simulink model "gm_uz_ssi_interface_2025b"  (R2025b)
settings: Solver=FixedStepDiscrete  StartTime=0.0  StopTime=0.005  RelTol=1e-3
undefined symbols (not defined in the file or in its folder): binary_or_gray, bit_sum, delay_first_clk_on_off, f_ADC, f_clock, PLL, ssi_clk_divider, ssi_encoder_bit_width_multi_turn, ssi_encoder_bit_width_single_turn, ssi_encoder_number_of_status_bits, t_ADC, t_clock, XData
libraries: hdlmdlgenlib x104, hdlsllib x90, simulink x33, simulink_extras x7
(part 1 of 4)
settings Model: Creator=micha  LastModifiedBy=micha
settings SolverCC: AlgebraicLoopSolver=TrustRegion
settings DataIOCC: LimitDataPoints=on  SaveOutput=off  SaveTime=off
settings OptimizationCC: BlockReduction=off  ConditionallyExecuteInputs=off  DefaultParameterBehavior=Inlined  InheritOutputTypeSmallerThanSingle=on  LifeSpan=inf
settings DebuggingCC: AlgebraicLoopMsg=error  ArtificialAlgebraicLoopMsg=none  InheritedTsInSrcMsg=none  SingleTaskRateTransMsg=error  UnconnectedInputMsg=warning  UnconnectedOutputMsg=warning  UnconnectedLineMsg=warning  AllowSymbolicDim=off  StrictBusMsg=ErrorOnBusTreatedAsVector  SFUnexpectedBacktrackingDiag=warning  SFNoUnconditionalDefaultTransitionDiag=warning  SFExecutionAtInitializationDiag=none  ArithmeticOperatorsInVariantConditions=warning
settings HardwareCC: ProdBitPerPointer=32.0  ProdBitPerSizeT=32.0  ProdBitPerPtrDiffT=32.0  ProdLargestAtomicFloat=None  ProdIntDivRoundTo=Undefined  ProdEndianess=Unspecified  ProdWordSize=32.0  ProdHWDeviceType=ASIC/FPGA->ASIC/FPGA  ProdEqTarget=off
settings ModelReferenceCC: EnableRefExpFcnMdlSchedulingChecks=on
settings SFSimCC: SimUseLocalCustomCode=off  CustomCodeUndefinedFunction=UseInterfaceOnly
settings RTWCC: RTWUseLocalCustomCode=off  GPUComputeCapability=3.5  DLArmComputeVersion=19.05
settings CodeAppCC: StateflowObjectComments=on
settings GRTTargetCC: TargetLangStandard=C89/C90 (ANSI)
settings ConfigComp: CovScope=ReferencedModels  CovMetricSettings=dw  CovSaveCumulativeToWorkspaceVar=on  CovSaveSingleToWorkspaceVar=on  CovExternalEMLEnable=off  CovSFcnEnable=off

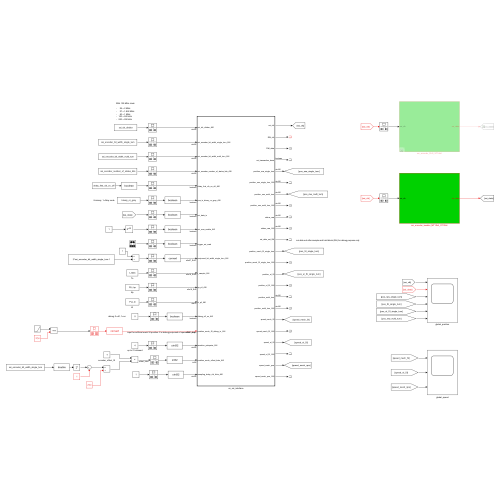
[thumbnail: Simulink's stored preview of the top-level diagram]
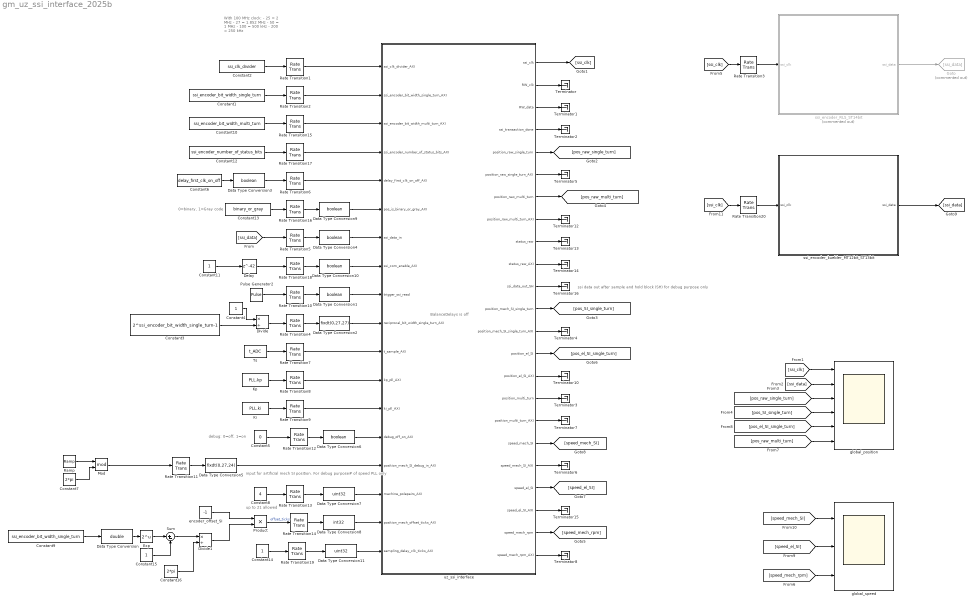
== system gm_uz_ssi_interface_2025b ==
  note: 0=binary, 1=Gray code
  note: With 100 MHz clock:
      |
      | -     25 = 2 MHz
      | -     27 = 1.852 MHz
      | -     50 = 1 MHz
      | -   100 = 500 kHz
      | -   200 = 250 kHz
  note: BalanceDelays is off
  note: debug: 0=off, 1=on
  note: up to 21 allowed
  note: ssi data out after sample and hold block (SH) for debug purpose only
  note: input for artificial mech SI position. For debug purpose# of speed PLL only
  Constant1 : Constant  Value=ssi_encoder_bit_width_single_turn  OutDataTypeStr=uint32  SampleTime=t_clock
  Constant10 : Constant  Value=ssi_encoder_bit_width_multi_turn  OutDataTypeStr=uint32  SampleTime=t_clock
  Constant{4,11,14..15} (4 alike) : Constant  SampleTime=t_clock
  Constant12 : Constant  Value=ssi_encoder_number_of_status_bits  OutDataTypeStr=uint32  SampleTime=t_clock
  Constant13 : Constant  Value=binary_or_gray  OutDataTypeStr=uint32  SampleTime=t_clock
  Constant16 : Constant  Value=2*pi  SampleTime=t_clock
  Constant2 : Constant  Value=ssi_clk_divider  OutDataTypeStr=uint32  SampleTime=t_clock
  Constant3 : Constant  Value=2^ssi_encoder_bit_width_single_turn-1  OutDataTypeStr=double  SampleTime=t_clock
  Constant5 : Constant  Value=0  SampleTime=t_clock
  Constant6 : Constant  Value=delay_first_clk_on_off  OutDataTypeStr=uint32  SampleTime=t_clock
  Constant7 : Constant  Value=2*pi  SampleTime=t_clock
  Constant8 : Constant  Value=4  SampleTime=t_clock
  Constant9 : Constant  Value=ssi_encoder_bit_width_single_turn  OutDataTypeStr=uint32  SampleTime=t_clock
  Data Type Conversion : DataTypeConversion  OutDataTypeStr=double  SaturateOnIntegerOverflow=off  RndMeth=Floor
  Data Type Conversion{1,3..4,6,9..10} (6 alike) : DataTypeConversion  OutDataTypeStr=boolean  SaturateOnIntegerOverflow=off  RndMeth=Floor
  Data Type Conversion11 : DataTypeConversion  OutDataTypeStr=uint32  SaturateOnIntegerOverflow=off  RndMeth=Floor
  Data Type Conversion2 : DataTypeConversion  OutDataTypeStr=fixdt(0,27,27)  SaturateOnIntegerOverflow=off  RndMeth=Floor
  Data Type Conversion5 : DataTypeConversion  OutDataTypeStr=fixdt(0,27,24)  SaturateOnIntegerOverflow=off  RndMeth=Floor
  Data Type Conversion7 : DataTypeConversion  OutDataTypeStr=uint32  SaturateOnIntegerOverflow=off  RndMeth=Floor
  Data Type Conversion8 : DataTypeConversion  OutDataTypeStr=int32  SaturateOnIntegerOverflow=off  RndMeth=Floor
  Delay : Delay  DelayLength=42
  Divide : Product  Inputs=*/
  Divide1 : Product  Inputs=*/
  Exp : Math  Operator=2^u
  Goto : Goto  Commented=on  GotoTag=ssi_data
  Ki : Constant  Value=PLL.ki  OutDataTypeStr=fixdt(0,18,0)  SampleTime=-1
  Kp : Constant  Value=PLL.kp  OutDataTypeStr=fixdt(0,18,5)  SampleTime=-1
  Mod : Math  Operator=mod
  Product : Product
  Pulse Generator2 : DiscretePulseGenerator  Period=f_clock/f_ADC  PulseWidth=0.04*f_clock/f_ADC  PhaseDelay=250  SampleTime=t_clock
  Ramp : simulink/Sources/Ramp  slope=2*pi*100  start=7.5e-5  InitialOutput=0
  Rate Transition{1..20} (20 alike) : RateTransition  OutPortSampleTime=t_clock
  Sum : Sum  Inputs=|+-
  Terminator{,1..8,10,12..16} (15 alike) : Terminator
  Ts : Constant  Value=t_ADC  OutDataTypeStr=fixdt(0,18,24)  SampleTime=-1
  encoder_offset_SI : Constant  Value=-1  SampleTime=t_clock
  global_position : Scope  NumInputPorts=6
      settings: ActiveDisplayYMinimum=-0.125  ActiveDisplayYMaximum=1.125  DataLoggingVariableName=ScopeData2
  global_speed : Scope  NumInputPorts=3
      settings: ActiveDisplayYMinimum=-40.08166  ActiveDisplayYMaximum=351.59007
  ssi_encoder_RLS_ST14bit : Subsystem  Commented=on
  ssi_encoder_kuebler_MT12bit_ST13bit : Subsystem
  uz_ssi_interface : Subsystem  TreatAsAtomicUnit=on
  wires:
  Data Type Conversion/1 -> Exp/1
  Divide1/1 -> Product/2
  Constant16/1 -> Divide1/2
  Sum/1 -> Divide1/1
  Exp/1 -> Sum/1
  Constant15/1 -> Sum/2
  Constant9/1 -> Data Type Conversion/1
  Product/1 -> Rate Transition14/1  "offset_ticks"
  uz_ssi_interface/17(position_multi_turn_AXI) -> Terminator7/1
  uz_ssi_interface/16(position_multi_turn) -> Terminator3/1
  ssi_encoder_kuebler_MT12bit_ST13bit/1(ssi_data) -> [ssi_data]
  Rate Transition20/1 -> ssi_encoder_kuebler_MT12bit_ST13bit/1(ssi_clk)
  [ssi_clk] -> Rate Transition20/1
  Constant14/1 -> Rate Transition19/1
  Rate Transition19/1 -> Data Type Conversion11/1
  Data Type Conversion11/1 -> uz_ssi_interface/18(sampling_delay_clk_ticks_AXI)
  [speed_el_SI] -> global_speed/2
  [speed_mech_SI] -> global_speed/1
  [pos_el_SI_single_turn] -> global_position/5
  [pos_raw_multi_turn] -> global_position/6
  [speed_mech_rpm] -> global_speed/3
  [ssi_clk] -> Rate Transition3/1
  Delay/1 -> Rate Transition18/1
  uz_ssi_interface/22(speed_mech_rpm) -> [speed_mech_rpm]
  uz_ssi_interface/11(ssi_data_out_SH) -> Terminator16/1
  uz_ssi_interface/12(position_mech_SI_single_turn) -> [pos_SI_single_turn]
  [pos_SI_single_turn] -> global_position/4
  [pos_raw_single_turn] -> global_position/3
  uz_ssi_interface/5(position_raw_single_turn) -> [pos_raw_single_turn]
  [ssi_data] -> global_position/2
  [ssi_clk] -> global_position/1
  uz_ssi_interface/20(speed_el_SI) -> [speed_el_SI]
  uz_ssi_interface/21(speed_el_SI_AXI) -> Terminator15/1
  uz_ssi_interface/10(status_raw_AXI) -> Terminator14/1
  uz_ssi_interface/9(status_raw) -> Terminator13/1
  uz_ssi_interface/8(position_raw_multi_turn_AXI) -> Terminator12/1
  uz_ssi_interface/7(position_raw_multi_turn) -> [pos_raw_multi_turn]
  Constant11/1 -> Delay/1
  Rate Transition18/1 -> Data Type Conversion10/1
  Data Type Conversion10/1 -> uz_ssi_interface/8(ssi_com_enable_AXI)
  Constant12/1 -> Rate Transition17/1
  Rate Transition17/1 -> uz_ssi_interface/4(ssi_encoder_number_of_status_bits_AXI)
  Data Type Conversion9/1 -> uz_ssi_interface/6(pos_is_binary_or_gray_AXI)
  Constant13/1 -> Rate Transition16/1
  Rate Transition16/1 -> Data Type Conversion9/1
  Constant10/1 -> Rate Transition15/1
  Rate Transition15/1 -> uz_ssi_interface/3(ssi_encoder_bit_width_multi_turn_AXI)
  uz_ssi_interface/15(position_el_SI_AXI) -> Terminator10/1
  uz_ssi_interface/14(position_el_SI) -> [pos_el_SI_single_turn]
  Data Type Conversion8/1 -> uz_ssi_interface/17(position_mech_offset_ticks_AXI)
  encoder_offset_SI/1 -> Product/1
  Rate Transition14/1 -> Data Type Conversion8/1
  Constant8/1 -> Rate Transition13/1
  Data Type Conversion7/1 -> uz_ssi_interface/16(machine_polepairs_AXI)
  Rate Transition13/1 -> Data Type Conversion7/1
  uz_ssi_interface/23(speed_mech_rpm_AXI) -> Terminator8/1
  Constant7/1 -> Mod/2
  Ramp/1 -> Mod/1
  Mod/1 -> Rate Transition11/1
  Constant5/1 -> Rate Transition12/1
  Rate Transition12/1 -> Data Type Conversion6/1
  Data Type Conversion6/1 -> uz_ssi_interface/14(debug_off_on_AXI)
  Data Type Conversion5/1 -> uz_ssi_interface/15(position_mech_SI_debug_in_AXI)
  Rate Transition11/1 -> Data Type Conversion5/1
  uz_ssi_interface/19(speed_mech_SI_AXI) -> Terminator6/1
  uz_ssi_interface/18(speed_mech_SI) -> [speed_mech_SI]
  Rate Transition9/1 -> uz_ssi_interface/13(ki_pll_AXI)
  Ki/1 -> Rate Transition9/1
  Rate Transition8/1 -> uz_ssi_interface/12(kp_pll_AXI)
  Kp/1 -> Rate Transition8/1
  Rate Transition7/1 -> uz_ssi_interface/11(t_sample_AXI)
  Ts/1 -> Rate Transition7/1
  uz_ssi_interface/13(position_mech_SI_single_turn_AXI) -> Terminator4/1
  Divide/1 -> Rate Transition4/1
  Constant4/1 -> Divide/1
  Data Type Conversion2/1 -> uz_ssi_interface/10(reciprocal_bit_width_single_turn_AXI)
  Rate Transition4/1 -> Data Type Conversion2/1
  Constant3/1 -> Divide/2
  Data Type Conversion4/1 -> uz_ssi_interface/7(ssi_data_in)
  Rate Transition5/1 -> Data Type Conversion4/1
  uz_ssi_interface/6(position_raw_single_turn_AXI) -> Terminator5/1
  Constant6/1 -> Data Type Conversion3/1
  Data Type Conversion3/1 -> Rate Transition6/1
  Rate Transition6/1 -> uz_ssi_interface/5(delay_first_clk_on_off_AXI)
  Data Type Conversion1/1 -> uz_ssi_interface/9(trigger_ssi_read)
  uz_ssi_interface/2(RW_clk) -> Terminator/1
  uz_ssi_interface/4(ssi_transaction_done) -> Terminator2/1
  uz_ssi_interface/3(RW_data) -> Terminator1/1
  uz_ssi_interface/1(ssi_clk) -> [ssi_clk]
  [ssi_data] -> Rate Transition5/1
  ssi_encoder_RLS_ST14bit/1(ssi_data) -> Goto/1
  Rate Transition3/1 -> ssi_encoder_RLS_ST14bit/1(ssi_clk)
  Rate Transition2/1 -> uz_ssi_interface/2(ssi_encoder_bit_width_single_turn_AXI)
  Constant1/1 -> Rate Transition2/1
  Rate Transition1/1 -> uz_ssi_interface/1(ssi_clk_divider_AXI)
  Constant2/1 -> Rate Transition1/1
  Pulse Generator2/1 -> Rate Transition10/1
  Rate Transition10/1 -> Data Type Conversion1/1

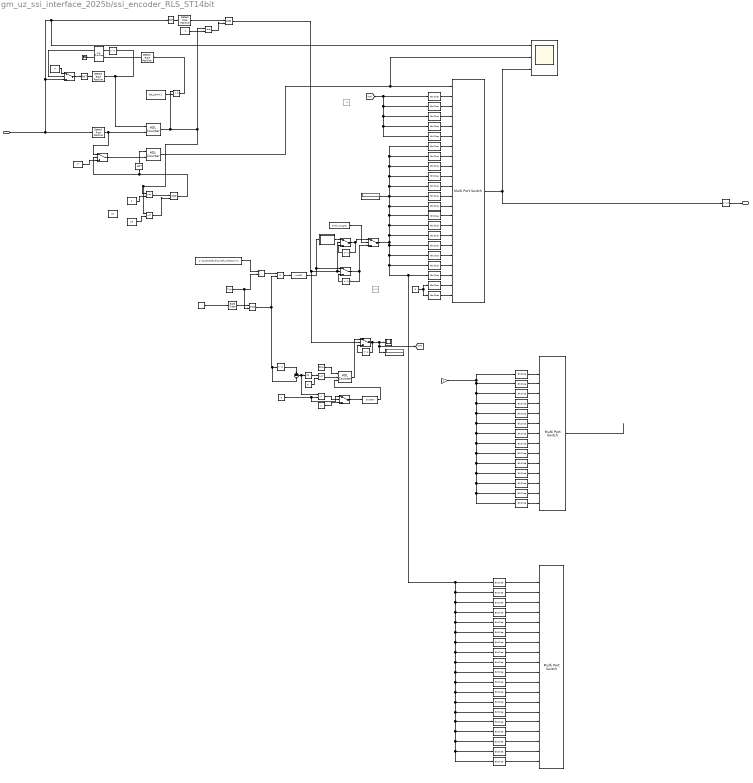
== system gm_uz_ssi_interface_2025b/ssi_encoder_RLS_ST14bit ==
  note: 19 bit single turn
  note: singleturn information
  note: Detect first falling edge of the clock
  note: 170 ns delay of the readhead
  note: multiturn information
  note: 14 bit single turn
  note: 5bit multiturn, 14bit single turn 2bit status
  ssi_clk : Inport
  AND : Logic  IconShape=distinctive  AllPortsSameDT=off  OutDataTypeStr=boolean
  AND1 : Logic  IconShape=distinctive  AllPortsSameDT=off  OutDataTypeStr=boolean
  Abs : Abs  SaturateOnIntegerOverflow=off
  Bit Slice{1,14,19,26,40} (5 alike) : hdlsllib/Logic and Bit Operations/Bit Slice  lidx=1  ridx=1
  Bit Slice10 : hdlsllib/Logic and Bit Operations/Bit Slice  lidx=5  ridx=5
  Bit Slice{11,16,23,37} (4 alike) : hdlsllib/Logic and Bit Operations/Bit Slice  lidx=4  ridx=4
  Bit Slice{12,17,24,38} (4 alike) : hdlsllib/Logic and Bit Operations/Bit Slice  lidx=3  ridx=3
  Bit Slice{13,18,25,39} (4 alike) : hdlsllib/Logic and Bit Operations/Bit Slice  lidx=2  ridx=2
  Bit Slice{15,20..21,27,41} (5 alike) : hdlsllib/Logic and Bit Operations/Bit Slice  lidx=0  ridx=0
  Bit Slice2 : hdlsllib/Logic and Bit Operations/Bit Slice  lidx=13  ridx=13
  Bit Slice22 : hdlsllib/Logic and Bit Operations/Bit Slice  lidx=5  ridx=5
  Bit Slice28 : hdlsllib/Logic and Bit Operations/Bit Slice  lidx=13  ridx=13
  Bit Slice29 : hdlsllib/Logic and Bit Operations/Bit Slice  lidx=12  ridx=12
  Bit Slice3 : hdlsllib/Logic and Bit Operations/Bit Slice  lidx=12  ridx=12
  Bit Slice30 : hdlsllib/Logic and Bit Operations/Bit Slice  lidx=11  ridx=11
  Bit Slice31 : hdlsllib/Logic and Bit Operations/Bit Slice  lidx=10  ridx=10
  Bit Slice32 : hdlsllib/Logic and Bit Operations/Bit Slice  lidx=9  ridx=9
  Bit Slice33 : hdlsllib/Logic and Bit Operations/Bit Slice  lidx=8  ridx=8
  Bit Slice34 : hdlsllib/Logic and Bit Operations/Bit Slice  lidx=7  ridx=7
  Bit Slice35 : hdlsllib/Logic and Bit Operations/Bit Slice  lidx=6  ridx=6
  Bit Slice36 : hdlsllib/Logic and Bit Operations/Bit Slice  lidx=5  ridx=5
  Bit Slice4 : hdlsllib/Logic and Bit Operations/Bit Slice  lidx=11  ridx=11
  Bit Slice42 : hdlsllib/Logic and Bit Operations/Bit Slice  lidx=13  ridx=13
  Bit Slice43 : hdlsllib/Logic and Bit Operations/Bit Slice  lidx=12  ridx=12
  Bit Slice44 : hdlsllib/Logic and Bit Operations/Bit Slice  lidx=11  ridx=11
  Bit Slice45 : hdlsllib/Logic and Bit Operations/Bit Slice  lidx=10  ridx=10
  Bit Slice46 : hdlsllib/Logic and Bit Operations/Bit Slice  lidx=9  ridx=9
  Bit Slice47 : hdlsllib/Logic and Bit Operations/Bit Slice  lidx=8  ridx=8
  Bit Slice48 : hdlsllib/Logic and Bit Operations/Bit Slice  lidx=7  ridx=7
  Bit Slice49 : hdlsllib/Logic and Bit Operations/Bit Slice  lidx=6  ridx=6
  Bit Slice5 : hdlsllib/Logic and Bit Operations/Bit Slice  lidx=10  ridx=10
  Bit Slice50 : hdlsllib/Logic and Bit Operations/Bit Slice  lidx=18  ridx=18
  Bit Slice51 : hdlsllib/Logic and Bit Operations/Bit Slice  lidx=17  ridx=17
  Bit Slice52 : hdlsllib/Logic and Bit Operations/Bit Slice  lidx=16  ridx=16
  Bit Slice53 : hdlsllib/Logic and Bit Operations/Bit Slice  lidx=15  ridx=15
  Bit Slice54 : hdlsllib/Logic and Bit Operations/Bit Slice  lidx=14  ridx=14
  Bit Slice6 : hdlsllib/Logic and Bit Operations/Bit Slice  lidx=9  ridx=9
  Bit Slice7 : hdlsllib/Logic and Bit Operations/Bit Slice  lidx=8  ridx=8
  Bit Slice8 : hdlsllib/Logic and Bit Operations/Bit Slice  lidx=7  ridx=7
  Bit Slice9 : hdlsllib/Logic and Bit Operations/Bit Slice  lidx=6  ridx=6
  Constant : Constant  Value=bit_sum+1  SampleTime=t_clock
  Constant1 : Constant  Value=0  SampleTime=t_clock
  Constant10 : Constant  Value=false  SampleTime=t_clock
  Constant11 : Constant  Value=0  SampleTime=t_clock
  Constant12 : Constant  SampleTime=t_clock
  Constant13 : Constant  Value=0  OutDataTypeStr=uint32  SampleTime=t_clock
  Constant14 : Constant  Commented=on  Value=19  OutDataTypeStr=uint32  SampleTime=t_clock
  Constant15 : Constant  Value=binary_or_gray  SampleTime=t_clock
  Constant16 : Constant  Value=15  SampleTime=t_clock
  Constant2 : Constant  SampleTime=t_clock
  Constant3 : Constant  Value=0  OutDataTypeStr=boolean  SampleTime=t_clock
  Constant4 : Constant  Value=5  SampleTime=t_clock
  Constant5 : Constant  Value=2  SampleTime=t_clock
  Constant6 : Constant  Commented=on  Value=3875  OutDataTypeStr=uint32  SampleTime=t_clock
  Constant7 : Constant  Value=2*pi  SampleTime=t_clock
  Constant8 : Constant  Value=22  SampleTime=t_clock
  Constant9 : Constant  Value=2^ssi_encoder_bit_width_single_turn-1  SampleTime=t_clock
  Data Type Conversion : DataTypeConversion  OutDataTypeStr=uint32  SaturateOnIntegerOverflow=off  RndMeth=Floor
  Data Type Conversion1 : DataTypeConversion  OutDataTypeStr=boolean  SaturateOnIntegerOverflow=off  RndMeth=Floor
  Delay : Delay  DelayLength=1
  Delay1 : Delay  DelayLength=17  SampleTime=t_clock
  Delay2 : Delay  DelayLength=1  SampleTime=t_clock
  Delay3 : Delay  DelayLength=1
  Delay4 : Delay  DelayLength=1  InitialCondition=19  SampleTime=t_clock
  Delay5 : Delay  DelayLength=1  SampleTime=t_clock
  Detect Rise Positive{,1..3} (4 alike) : simulink/Logic and Bit Operations/Detect Rise Positive  vinit=0  OutDataTypeStr=boolean
  Display : Display
  Display1 : Display
  Divide : Product  Inputs=*/
  Gain : Gain
  HDL Counter : hdlsllib/Sources/HDL Counter  CountType=Count limited  CountInit=0  CountStep=1  CountMax=bit_sum+1  CountFromType=Initial value  CountFrom=0  CountResetPort=on  CountLoadPort=off  CountEnbPort=on  CountDirPort=off  CountHitOutputPort=off  CountDataType=Unsigned  CountWordLen=8  CountFracLen=0  CountSampTime=t_clock
  HDL Counter1 : hdlsllib/Sources/HDL Counter  CountType=Count limited  CountInit=0  CountStep=1  CountMax=bit_sum+1  CountFromType=Initial value  CountFrom=0  CountResetPort=on  CountLoadPort=off  CountEnbPort=on  CountDirPort=off  CountHitOutputPort=off  CountDataType=Unsigned  CountWordLen=8  CountFracLen=0  CountSampTime=t_clock
  HDL Counter2 : hdlsllib/Sources/HDL Counter  CountType=Count limited  CountInit=19  CountStep=1  CountMax=ssi_encoder_bit_width_multi_turn  CountFromType=Initial value  CountFrom=19  CountResetPort=on  CountLoadPort=off  CountEnbPort=on  CountDirPort=on  CountHitOutputPort=off  CountDataType=Unsigned  CountWordLen=5  CountFracLen=0  CountSampTime=t_clock
  Index Vector : MultiPortSwitch  DataPortOrder=Zero-based contiguous  Inputs=21  zeroidx=on  SaturateOnIntegerOverflow=off  InputSameDT=off
  Index Vector1 : MultiPortSwitch  DataPortOrder=Zero-based contiguous  Inputs=14  zeroidx=on  SaturateOnIntegerOverflow=off  InputSameDT=off
  Index Vector2 : MultiPortSwitch  DataPortOrder=Zero-based contiguous  Inputs=19  zeroidx=on  SaturateOnIntegerOverflow=off  InputSameDT=off
  MATLAB Function : MATLAB Function  TreatAsAtomicUnit=on
  Mod : Math  Operator=mod
  NOT : Logic  Operator=NOT  IconShape=distinctive  AllPortsSameDT=off  OutDataTypeStr=boolean
  NOT1 : Logic  Operator=NOT  IconShape=distinctive  AllPortsSameDT=off  OutDataTypeStr=boolean
  NOT2 : Logic  Operator=NOT  IconShape=distinctive  AllPortsSameDT=off  OutDataTypeStr=boolean
  Product : Product
  Ramp : simulink/Sources/Ramp  slope=-2*pi*50  start=7.5e-5  InitialOutput=0
  Rate Transition : RateTransition  OutPortSampleTime=t_clock
  Relational Operator : RelationalOperator  OutDataTypeStr=boolean  RndMeth=Simplest  InputSameDT=off
  Relational Operator1 : RelationalOperator  OutDataTypeStr=boolean  RndMeth=Simplest  InputSameDT=off
  Relational Operator2 : RelationalOperator  Operator===  OutDataTypeStr=boolean  RndMeth=Simplest  InputSameDT=off
  Relational Operator3 : RelationalOperator  Operator=<=  OutDataTypeStr=boolean  RndMeth=Simplest  InputSameDT=off
  Relational Operator4 : RelationalOperator  OutDataTypeStr=boolean  RndMeth=Simplest  InputSameDT=off
  Relational Operator5 : RelationalOperator  Operator=<  OutDataTypeStr=boolean  RndMeth=Simplest  InputSameDT=off
  S-R Flip-Flop : simulink_extras/Flip Flops/S-R Flip-Flop  initial_condition=0
  Scope : Scope  NumInputPorts=3
      settings: ActiveDisplayYMinimum=-2.5  ActiveDisplayYMaximum=22.5
  Scope1 : Scope
  Sum : Sum  Inputs=+-
  Switch{,1..6} (7 alike) : Switch  Criteria=u2 > Threshold  SaturateOnIntegerOverflow=off  InputSameDT=off
  Terminator : Terminator
  ssi_data : Outport
  wires:
  Gain/1 -> Bit Slice29/1, Bit Slice30/1, Bit Slice31/1, Bit Slice32/1, Bit Slice33/1, Bit Slice34/1, Bit Slice35/1, Bit Slice22/1, Bit Slice23/1, Bit Slice24/1, Bit Slice25/1, Bit Slice26/1, Bit Slice27/1, Bit Slice28/1
  Index Vector/1 -> Delay1/1, Scope/3
  Switch5/1 -> Bit Slice11/1, Bit Slice10/1, Bit Slice9/1, Bit Slice8/1, Bit Slice7/1, Bit Slice3/1, Bit Slice2/1, Bit Slice4/1, Bit Slice5/1, Bit Slice6/1, Display/1, Bit Slice12/1, Bit Slice13/1, Bit Slice14/1, Bit Slice15/1, Bit Slice50/1, Bit Slice51/1, Bit Slice52/1, Bit Slice53/1, Bit Slice54/1, Bit Slice42/1, Bit Slice43/1, Bit Slice44/1, Bit Slice45/1, Bit Slice46/1, Bit Slice47/1, Bit Slice48/1, Bit Slice49/1, Bit Slice36/1, Bit Slice41/1, Bit Slice40/1, Bit Slice39/1, Bit Slice38/1, Bit Slice37/1
  Bit Slice51/1 -> Index Vector2/3
  Bit Slice54/1 -> Index Vector2/6
  Bit Slice50/1 -> Index Vector2/2
  Bit Slice53/1 -> Index Vector2/5
  Bit Slice52/1 -> Index Vector2/4
  Bit Slice39/1 -> Index Vector2/18
  Bit Slice49/1 -> Index Vector2/14
  Bit Slice43/1 -> Index Vector2/8
  Bit Slice48/1 -> Index Vector2/13
  Bit Slice46/1 -> Index Vector2/11
  Bit Slice45/1 -> Index Vector2/10
  Bit Slice38/1 -> Index Vector2/17
  Bit Slice42/1 -> Index Vector2/7
  Bit Slice41/1 -> Index Vector2/20
  Bit Slice44/1 -> Index Vector2/9
  Bit Slice36/1 -> Index Vector2/15
  Bit Slice40/1 -> Index Vector2/19
  Bit Slice37/1 -> Index Vector2/16
  Bit Slice47/1 -> Index Vector2/12
  Index Vector1/1 -> ?
  Bit Slice24/1 -> Index Vector1/12
  Bit Slice25/1 -> Index Vector1/13
  Bit Slice32/1 -> Index Vector1/6
  Bit Slice30/1 -> Index Vector1/4
  Bit Slice35/1 -> Index Vector1/9
  Bit Slice27/1 -> Index Vector1/15
  Bit Slice31/1 -> Index Vector1/5
  Bit Slice23/1 -> Index Vector1/11
  Bit Slice34/1 -> Index Vector1/8
  Bit Slice28/1 -> Index Vector1/2
  Bit Slice22/1 -> Index Vector1/10
  Bit Slice26/1 -> Index Vector1/14
  Bit Slice33/1 -> Index Vector1/7
  Bit Slice29/1 -> Index Vector1/3
  Delay5/1 -> Switch6/3
  Switch6/1 -> Switch5/1, Delay5/1
  MATLAB Function/1(y) -> Switch6/1
  Switch1/1 -> Switch5/3, Delay2/1
  Constant15/1 -> Switch5/2
  Data Type Conversion1/1 -> HDL Counter2/3
  Constant13/1 -> Bit Slice21/1, Bit Slice1/1
  Bit Slice21/1 -> Index Vector/22
  Bit Slice1/1 -> Index Vector/21
  Bit Slice15/1 -> Index Vector/20
  Bit Slice14/1 -> Index Vector/19
  Bit Slice13/1 -> Index Vector/18
  Bit Slice12/1 -> Index Vector/17
  Bit Slice11/1 -> Index Vector/16
  Bit Slice10/1 -> Index Vector/15
  Bit Slice9/1 -> Index Vector/14
  Bit Slice8/1 -> Index Vector/13
  Bit Slice7/1 -> Index Vector/12
  Bit Slice6/1 -> Index Vector/11
  Bit Slice5/1 -> Index Vector/10
  Bit Slice4/1 -> Index Vector/9
  Bit Slice3/1 -> Index Vector/8
  Bit Slice2/1 -> Index Vector/7
  Bit Slice20/1 -> Index Vector/6
  Bit Slice19/1 -> Index Vector/5
  Bit Slice18/1 -> Index Vector/4
  Bit Slice17/1 -> Index Vector/3
  Bit Slice16/1 -> Index Vector/2
  [MT] -> Bit Slice16/1, Bit Slice20/1, Bit Slice19/1, Bit Slice18/1, Bit Slice17/1
  Constant12/1 -> Switch4/3
  Switch4/1 -> Data Type Conversion1/1
  Relational Operator5/1 -> Switch4/2
  Constant11/1 -> Relational Operator5/2, Switch4/1
  Constant10/1 -> HDL Counter2/1
  Switch2/1 -> Delay4/1, Scope1/1, Display1/1, [MT]
  Delay4/1 -> Switch2/3
  HDL Counter2/1 -> Switch2/1
  Relational Operator4/1 -> HDL Counter2/2
  Constant4/1 -> Relational Operator4/2
  Abs/1 -> Relational Operator4/1
  Sum/1 -> Abs/1, Relational Operator5/1
  Mod/1 -> Product/2, Delay3/1, Sum/2
  Delay3/1 -> Sum/1
  Delay1/1 -> ssi_data/1
  HDL Counter1/1 -> Index Vector/1, Scope/2
  Constant3/1 -> Switch3/3
  AND/1 -> Switch1/2, Switch6/2, Switch2/2
  Data Type Conversion/1 -> MATLAB Function/1(u), Switch1/1
  Delay2/1 -> Switch1/3
  Rate Transition/1 -> Mod/1
  Product/1 -> Data Type Conversion/1
  Constant7/1 -> Divide/2, Mod/2
  Divide/1 -> Product/1
  Constant9/1 -> Divide/1
  Ramp/1 -> Rate Transition/1
  NOT2/1 -> HDL Counter1/1
  Switch3/1 -> HDL Counter1/2
  Constant16/1 -> Relational Operator3/2
  Relational Operator3/1 -> AND1/2
  Constant5/1 -> Relational Operator1/2
  AND1/1 -> Switch3/2, NOT2/1
  Relational Operator1/1 -> AND1/1
  ssi_clk/1 -> Detect Rise Positive1/1, Switch/3, NOT1/1, Scope/1
  Constant1/1 -> Switch/1
  S-R Flip-Flop/2 -> Terminator/1
  HDL Counter/1 -> Relational Operator/1, Relational Operator2/1, Relational Operator1/1, Relational Operator3/1
  Detect Rise Positive1/1 -> Switch3/1, HDL Counter/2
  Detect Rise Positive3/1 -> AND/1
  NOT1/1 -> Detect Rise Positive3/1
  Constant2/1 -> Relational Operator2/2
  Relational Operator2/1 -> AND/2
  Detect Rise Positive/1 -> Delay/1, HDL Counter/1
  Detect Rise Positive2/1 -> S-R Flip-Flop/2
  Relational Operator/1 -> Detect Rise Positive2/1
  Delay/1 -> S-R Flip-Flop/1
  S-R Flip-Flop/1 -> Switch/2
  Switch/1 -> NOT/1
  Constant/1 -> Relational Operator/2
  NOT/1 -> Detect Rise Positive/1

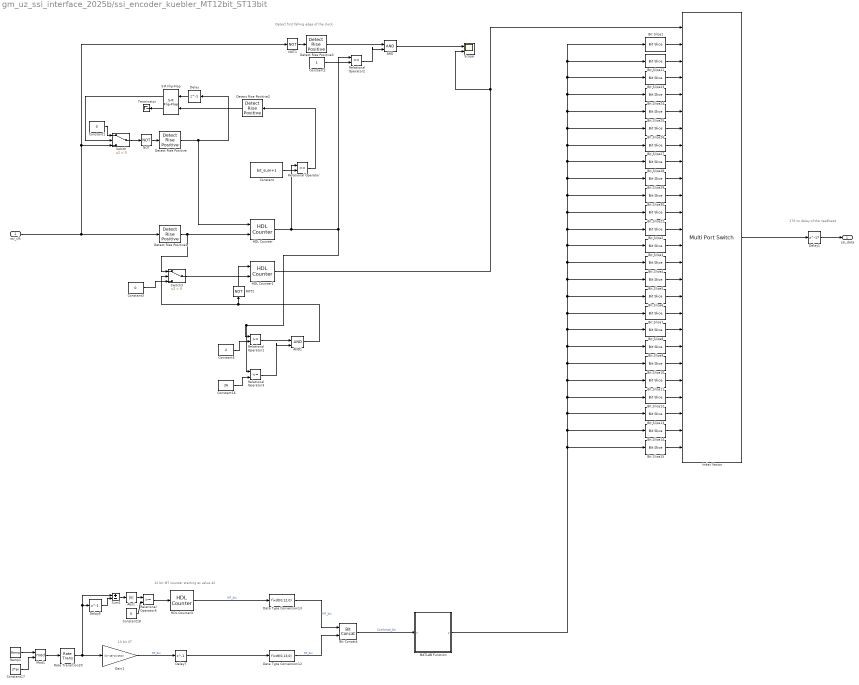
== system gm_uz_ssi_interface_2025b/ssi_encoder_kuebler_MT12bit_ST13bit ==
  note: 13 bit ST
  note: Detect first falling edge of the clock
  note: 170 ns delay of the readhead
  note: 12 bit MT counter starting at value 42
  ssi_clk : Inport
  AND : Logic  IconShape=distinctive  AllPortsSameDT=off  OutDataTypeStr=boolean
  AND1 : Logic  IconShape=distinctive  AllPortsSameDT=off  OutDataTypeStr=boolean
  Abs1 : Abs  SaturateOnIntegerOverflow=off
  Bit Concat4 : hdlsllib/Logic and Bit Operations/Bit Concat  numInputs=2
  Bit Slice1 : hdlsllib/Logic and Bit Operations/Bit Slice  lidx=24  ridx=24
  Bit Slice10 : hdlsllib/Logic and Bit Operations/Bit Slice  lidx=5  ridx=5
  Bit Slice11 : hdlsllib/Logic and Bit Operations/Bit Slice  lidx=4  ridx=4
  Bit Slice12 : hdlsllib/Logic and Bit Operations/Bit Slice  lidx=3  ridx=3
  Bit Slice13 : hdlsllib/Logic and Bit Operations/Bit Slice  lidx=2  ridx=2
  Bit Slice14 : hdlsllib/Logic and Bit Operations/Bit Slice  lidx=1  ridx=1
  Bit Slice15 : hdlsllib/Logic and Bit Operations/Bit Slice  lidx=0  ridx=0
  Bit Slice2 : hdlsllib/Logic and Bit Operations/Bit Slice  lidx=13  ridx=13
  Bit Slice21 : hdlsllib/Logic and Bit Operations/Bit Slice  lidx=23  ridx=23
  Bit Slice22 : hdlsllib/Logic and Bit Operations/Bit Slice  lidx=14  ridx=14
  Bit Slice23 : hdlsllib/Logic and Bit Operations/Bit Slice  lidx=22  ridx=22
  Bit Slice24 : hdlsllib/Logic and Bit Operations/Bit Slice  lidx=21  ridx=21
  Bit Slice25 : hdlsllib/Logic and Bit Operations/Bit Slice  lidx=20  ridx=20
  Bit Slice26 : hdlsllib/Logic and Bit Operations/Bit Slice  lidx=19  ridx=19
  Bit Slice27 : hdlsllib/Logic and Bit Operations/Bit Slice  lidx=18  ridx=18
  Bit Slice28 : hdlsllib/Logic and Bit Operations/Bit Slice  lidx=17  ridx=17
  Bit Slice29 : hdlsllib/Logic and Bit Operations/Bit Slice  lidx=16  ridx=16
  Bit Slice3 : hdlsllib/Logic and Bit Operations/Bit Slice  lidx=12  ridx=12
  Bit Slice30 : hdlsllib/Logic and Bit Operations/Bit Slice  lidx=15  ridx=15
  Bit Slice4 : hdlsllib/Logic and Bit Operations/Bit Slice  lidx=11  ridx=11
  Bit Slice5 : hdlsllib/Logic and Bit Operations/Bit Slice  lidx=10  ridx=10
  Bit Slice6 : hdlsllib/Logic and Bit Operations/Bit Slice  lidx=9  ridx=9
  Bit Slice7 : hdlsllib/Logic and Bit Operations/Bit Slice  lidx=8  ridx=8
  Bit Slice8 : hdlsllib/Logic and Bit Operations/Bit Slice  lidx=7  ridx=7
  Bit Slice9 : hdlsllib/Logic and Bit Operations/Bit Slice  lidx=6  ridx=6
  Constant : Constant  Value=bit_sum+1  SampleTime=t_clock
  Constant1 : Constant  Value=0  SampleTime=t_clock
  Constant16 : Constant  Value=26  SampleTime=t_clock
  Constant17 : Constant  Value=2*pi  SampleTime=t_clock
  Constant18 : Constant  Value=5  SampleTime=t_clock
  Constant2 : Constant  SampleTime=t_clock
  Constant3 : Constant  Value=0  OutDataTypeStr=boolean  SampleTime=t_clock
  Constant5 : Constant  Value=2  SampleTime=t_clock
  Data Type Conversion12 : DataTypeConversion  OutDataTypeStr=fixdt(0,13,0)  SaturateOnIntegerOverflow=off  RndMeth=Floor
  Data Type Conversion13 : DataTypeConversion  OutDataTypeStr=fixdt(0,12,0)  SaturateOnIntegerOverflow=off  RndMeth=Floor
  Delay : Delay  DelayLength=1
  Delay1 : Delay  DelayLength=17  SampleTime=t_clock
  Delay6 : Delay  DelayLength=1
  Delay7 : Delay  DelayLength=1
  Detect Rise Positive{,1..3} (4 alike) : simulink/Logic and Bit Operations/Detect Rise Positive  vinit=0  OutDataTypeStr=boolean
  Gain1 : Gain  Gain=((2^13)-1)/(2*pi)  OutDataTypeStr=uint32
  HDL Counter : hdlsllib/Sources/HDL Counter  CountType=Count limited  CountInit=0  CountStep=1  CountMax=bit_sum+1  CountFromType=Initial value  CountFrom=0  CountResetPort=on  CountLoadPort=off  CountEnbPort=on  CountDirPort=off  CountHitOutputPort=off  CountDataType=Unsigned  CountWordLen=8  CountFracLen=0  CountSampTime=t_clock
  HDL Counter1 : hdlsllib/Sources/HDL Counter  CountType=Count limited  CountInit=0  CountStep=1  CountMax=bit_sum+1  CountFromType=Initial value  CountFrom=0  CountResetPort=on  CountLoadPort=off  CountEnbPort=on  CountDirPort=off  CountHitOutputPort=off  CountDataType=Unsigned  CountWordLen=8  CountFracLen=0  CountSampTime=t_clock
  HDL Counter3 : hdlsllib/Sources/HDL Counter  CountType=Count limited  CountInit=42  CountStep=1  CountMax=4095  CountFromType=Initial value  CountFrom=42  CountResetPort=off  CountLoadPort=off  CountEnbPort=on  CountDirPort=off  CountHitOutputPort=off  CountDataType=Unsigned  CountWordLen=12  CountFracLen=0  CountSampTime=1
  Index Vector : MultiPortSwitch  DataPortOrder=Zero-based contiguous  Inputs=25  zeroidx=on  SaturateOnIntegerOverflow=off  InputSameDT=off
  MATLAB Function : MATLAB Function  TreatAsAtomicUnit=on
  Mod1 : Math  Operator=mod
  NOT : Logic  Operator=NOT  IconShape=distinctive  AllPortsSameDT=off  OutDataTypeStr=boolean
  NOT1 : Logic  Operator=NOT  IconShape=distinctive  AllPortsSameDT=off  OutDataTypeStr=boolean
  NOT2 : Logic  Operator=NOT  IconShape=distinctive  AllPortsSameDT=off  OutDataTypeStr=boolean
  Ramp1 : simulink/Sources/Ramp  slope=2*pi*50  start=0  InitialOutput=0
  Rate Transition20 : RateTransition  OutPortSampleTime=t_clock
  Relational Operator : RelationalOperator  OutDataTypeStr=boolean  RndMeth=Simplest  InputSameDT=off
  Relational Operator1 : RelationalOperator  OutDataTypeStr=boolean  RndMeth=Simplest  InputSameDT=off
  Relational Operator2 : RelationalOperator  Operator===  OutDataTypeStr=boolean  RndMeth=Simplest  InputSameDT=off
  Relational Operator3 : RelationalOperator  Operator=<=  OutDataTypeStr=boolean  RndMeth=Simplest  InputSameDT=off
  Relational Operator6 : RelationalOperator  OutDataTypeStr=boolean  RndMeth=Simplest  InputSameDT=off
  S-R Flip-Flop : simulink_extras/Flip Flops/S-R Flip-Flop  initial_condition=0
  Scope : Scope  NumInputPorts=2
      settings: ActiveDisplayYMinimum=-0.125  ActiveDisplayYMaximum=1.125
  Sum1 : Sum  Inputs=+-
  Switch : Switch  Criteria=u2 > Threshold  SaturateOnIntegerOverflow=off  InputSameDT=off
  Switch3 : Switch  Criteria=u2 > Threshold  SaturateOnIntegerOverflow=off  InputSameDT=off
  Terminator : Terminator
  ssi_data : Outport
  wires:
  MATLAB Function/1(y) -> Bit Slice12/1, Bit Slice9/1, Bit Slice1/1, Bit Slice21/1, Bit Slice23/1, Bit Slice24/1, Bit Slice25/1, Bit Slice26/1, Bit Slice27/1, Bit Slice28/1, Bit Slice29/1, Bit Slice30/1, Bit Slice22/1, Bit Slice2/1, Bit Slice3/1, Bit Slice4/1, Bit Slice5/1, Bit Slice6/1, Bit Slice7/1, Bit Slice8/1, Bit Slice10/1, Bit Slice11/1, Bit Slice13/1, Bit Slice14/1, Bit Slice15/1
  Bit Concat4/1 -> MATLAB Function/1(u)  "Combined_bin"
  Bit Slice1/1 -> Index Vector/2
  Bit Slice21/1 -> Index Vector/3
  Bit Slice12/1 -> Index Vector/23
  Bit Slice11/1 -> Index Vector/22
  Bit Slice29/1 -> Index Vector/10
  Bit Slice13/1 -> Index Vector/24
  Bit Slice30/1 -> Index Vector/11
  Bit Slice7/1 -> Index Vector/18
  Bit Slice10/1 -> Index Vector/21
  Bit Slice4/1 -> Index Vector/15
  Bit Slice28/1 -> Index Vector/9
  Bit Slice25/1 -> Index Vector/6
  Bit Slice14/1 -> Index Vector/25
  Bit Slice27/1 -> Index Vector/8
  Bit Slice15/1 -> Index Vector/26
  Bit Slice22/1 -> Index Vector/12
  Bit Slice23/1 -> Index Vector/4
  Bit Slice26/1 -> Index Vector/7
  Bit Slice24/1 -> Index Vector/5
  Bit Slice8/1 -> Index Vector/19
  Bit Slice3/1 -> Index Vector/14
  Bit Slice9/1 -> Index Vector/20
  Bit Slice2/1 -> Index Vector/13
  Bit Slice5/1 -> Index Vector/16
  Bit Slice6/1 -> Index Vector/17
  AND/1 -> Scope/1
  Index Vector/1 -> Delay1/1
  HDL Counter1/1 -> Scope/2, Index Vector/1
  Relational Operator6/1 -> HDL Counter3/1
  Data Type Conversion13/1 -> Bit Concat4/1  "MT_bin"
  Rate Transition20/1 -> Gain1/1, Delay6/1, Sum1/1
  Delay7/1 -> Data Type Conversion12/1
  Sum1/1 -> Abs1/1
  Abs1/1 -> Relational Operator6/1
  Mod1/1 -> Rate Transition20/1
  Constant18/1 -> Relational Operator6/2
  Data Type Conversion12/1 -> Bit Concat4/2  "ST_bin"
  Gain1/1 -> Delay7/1  "ST_bin"
  Ramp1/1 -> Mod1/1
  HDL Counter3/1 -> Data Type Conversion13/1  "MT_bin"
  Delay6/1 -> Sum1/2
  Constant17/1 -> Mod1/2
  Delay1/1 -> ssi_data/1
  Constant3/1 -> Switch3/3
  NOT2/1 -> HDL Counter1/1
  Switch3/1 -> HDL Counter1/2
  Constant16/1 -> Relational Operator3/2
  Relational Operator3/1 -> AND1/2
  Constant5/1 -> Relational Operator1/2
  AND1/1 -> Switch3/2, NOT2/1
  Relational Operator1/1 -> AND1/1
  ssi_clk/1 -> Detect Rise Positive1/1, Switch/3, NOT1/1
  Constant1/1 -> Switch/1
  S-R Flip-Flop/2 -> Terminator/1
  HDL Counter/1 -> Relational Operator/1, Relational Operator2/1, Relational Operator1/1, Relational Operator3/1
  Detect Rise Positive1/1 -> Switch3/1, HDL Counter/2
  Detect Rise Positive3/1 -> AND/1
  NOT1/1 -> Detect Rise Positive3/1
  Constant2/1 -> Relational Operator2/2
  Relational Operator2/1 -> AND/2
  Detect Rise Positive/1 -> Delay/1, HDL Counter/1
  Detect Rise Positive2/1 -> S-R Flip-Flop/2
  Relational Operator/1 -> Detect Rise Positive2/1
  Delay/1 -> S-R Flip-Flop/1
  S-R Flip-Flop/1 -> Switch/2
  Switch/1 -> NOT/1
  Constant/1 -> Relational Operator/2
  NOT/1 -> Detect Rise Positive/1
